simulink model "Prac03_2_1"  (R2015a)
settings: Solver=ode45  StartTime=0.0  StopTime=8  RelTol=1e-3
libraries: dspsigops x2, simulink x1
settings Model: Creator=Josemi  LastModifiedBy=Josemi

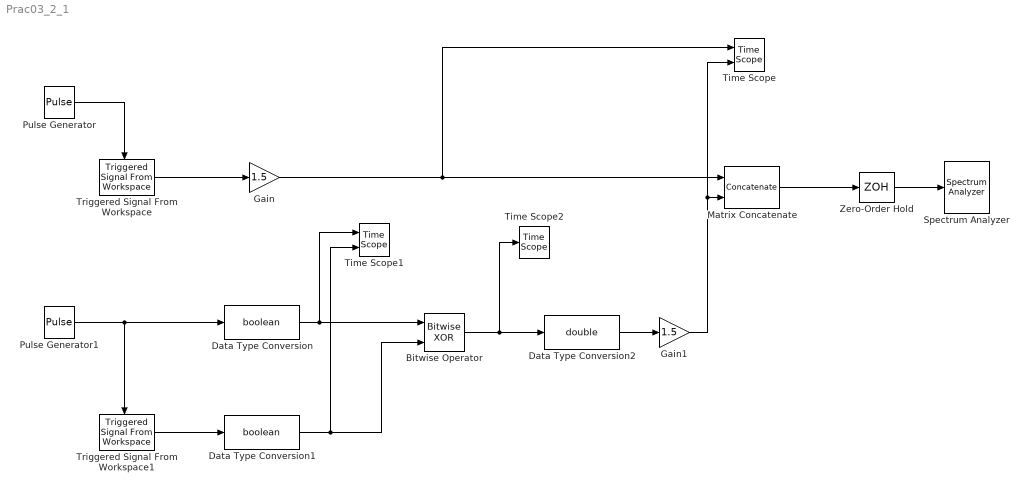
== system Prac03_2_1 ==
  Bitwise Operator : simulink/Logic and Bit Operations/Bitwise Operator  logicop=XOR  UseBitMask=off  NumInputPorts=2  BitMask=bin2dec('11011001')  BitMaskRealWorld=Stored Integer
  Data Type Conversion : DataTypeConversion  OutDataTypeStr=boolean
  Data Type Conversion1 : DataTypeConversion  OutDataTypeStr=boolean
  Data Type Conversion2 : DataTypeConversion  OutDataTypeStr=double
  Gain : Gain  Gain=1.5
  Gain1 : Gain  Gain=1.5
  Matrix Concatenate : Concatenate  Mode=Multidimensional array  ConcatenateDimension=2
  Pulse Generator : DiscretePulseGenerator  PulseType=Time based  Amplitude=0.5  Period=0.5  PulseWidth=50
  Pulse Generator1 : DiscretePulseGenerator  PulseType=Time based  Amplitude=0.5  Period=0.5  PulseWidth=50
  Spectrum Analyzer : SpectrumAnalyzer
  Time Scope : TimeScope  DefaultConfigurationName=spbscopes.TimeScopeBlockCfg  NumInputPorts=2
  Time Scope1 : TimeScope  DefaultConfigurationName=spbscopes.TimeScopeBlockCfg  NumInputPorts=2
  Time Scope2 : TimeScope  DefaultConfigurationName=spbscopes.TimeScopeBlockCfg
  Triggered Signal From Workspace : dspsigops/Triggered Signal From Workspace  Signal=[1 0 1 0 0 0 1 1 1 0 1 1 0 0 0]  TriggerType=Rising edge  ic=0  SamplesPerFrame=1  OutputAfterFinalValue=Setting to zero
  Triggered Signal From Workspace1 : dspsigops/Triggered Signal From Workspace  Signal=[1 0 1 0 0 0 1 1 1 0 1 1 0 0 0]  TriggerType=Rising edge  ic=0  SamplesPerFrame=1  OutputAfterFinalValue=Setting to zero
  Zero-Order Hold : ZeroOrderHold  SampleTime=0.0025
  wires:
  Pulse Generator/1 -> Triggered Signal From Workspace/Trigger
  Pulse Generator1/1 -> Triggered Signal From Workspace1/Trigger, Data Type Conversion/1
  Triggered Signal From Workspace/1 -> Gain/1
  Triggered Signal From Workspace1/1 -> Data Type Conversion1/1
  Data Type Conversion/1 -> Time Scope1/1, Bitwise Operator/1
  Data Type Conversion1/1 -> Time Scope1/2, Bitwise Operator/2
  Bitwise Operator/1 -> Time Scope2/1, Data Type Conversion2/1
  Data Type Conversion2/1 -> Gain1/1
  Gain/1 -> Time Scope/1, Matrix Concatenate/1
  Gain1/1 -> Time Scope/2, Matrix Concatenate/2
  Zero-Order Hold/1 -> Spectrum Analyzer/1
  Matrix Concatenate/1 -> Zero-Order Hold/1
